simulink model "torqueBalancing"  (Simulink 8.6)
settings: Solver=FixedStepDiscrete  StartTime=0.0  StopTime=simulationTime  FixedStep=Ts  RelTol=1e-3
InitFcn:
  | initTorqueBalancing;
values from neighbouring files (symbols this model uses):
  DEMO_MOVEMENTS = false    [initTorqueBalancing.m]
  LEFT_RIGHT_FOOT_IN_CONTACT = [1 1]    [initTorqueBalancing.m]
  ON_GAZEBO = false    [initTorqueBalancing.m]
  SMOOTH_DES_COM = 1    [initTorqueBalancing.m]
  SMOOTH_DES_Q = 1    [initTorqueBalancing.m]
  Ts = 0.01    [initTorqueBalancing.m]
  USE_QP_SOLVER = 0    [initTorqueBalancing.m]
  USE_SM = true    [initTorqueBalancing.m]
  WBT_modelName = 'matlabTorqueBalancing'    [initTorqueBalancing.m]
undefined symbols (not defined in the file or in its folder): bVectorConstraints, ConstraintsMatrix, DiscIntNeverNeededParam, gain, impedencesSat, reg, ROBOT_DOF, ROBOT_DOF_FOR_SIMULINK, sat, sm
libraries: WBToolboxLibrary x55, WBCLibrary x2, simulink x2
(part 1 of 2)
settings Model: Creator=daniele  LastModifiedBy=DanielePucci
settings DataIOCC: SignalLoggingSaveFormat=Dataset
settings DebuggingCC: FcnCallInpInsideContextMsg=EnableAllAsWarning
settings SFSimCC: SimParseCustomCode=off
settings ConfigComp: CovSFcnEnable=off

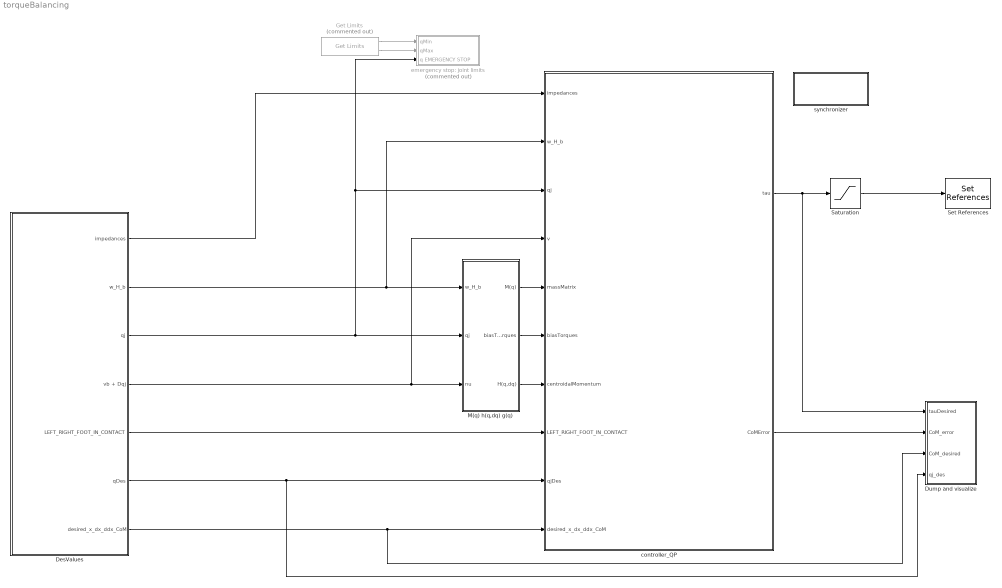
== system torqueBalancing ==
  DesValues : Subsystem  Priority=-10
  Dump and visualize : Subsystem
  Get Limits : WBToolboxLibrary/wholeBodyStates/Get Limits  Commented=on  limitsType=Position  robotName=WBT_robotName  localName=WBT_modelName  wbiFile=WBT_wbiFilename  wbiList=WBT_wbiList
  M(q) h(q,dq) g(q) : Subsystem
  Saturation : Saturate  UpperLimit=sat.torque  LowerLimit=-sat.torque
  Set References : WBToolboxLibrary/wholeBodyActuators/Set References  controlType=Torque  robotName=WBT_robotName  localName=WBT_modelName  wbiFile=WBT_wbiFilename  wbiList=WBT_wbiList
  controller_QP : Subsystem
  emergency stop: joint limits : Subsystem  Commented=on
  synchronizer : Subsystem
      mask Display: disp('SYNCHRONIZER')
  wires:
  M(q) h(q,dq) g(q)/1(M(q)) -> controller_QP/5(massMatrix)
  Get Limits/1 -> emergency stop: joint limits/1(qMin)
  Get Limits/2 -> emergency stop: joint limits/2(qMax)
  DesValues/3(qj) -> emergency stop: joint limits/3(q EMERGENCY STOP), controller_QP/3(qj), M(q) h(q,dq) g(q)/2(qj)
  M(q) h(q,dq) g(q)/2(biasTorques) -> controller_QP/6(biasTorques)
  M(q) h(q,dq) g(q)/3(H(q,dq)) -> controller_QP/7(centroidalMomentum)
  controller_QP/1("tau ") -> Saturation/1, Dump and visualize/1(tauDesired)
  controller_QP/2(CoMError) -> Dump and visualize/2(CoM_error)
  DesValues/6(qDes) -> Dump and visualize/4(qj_des), controller_QP/9(qjDes)
  DesValues/5(LEFT_RIGHT_FOOT_IN_CONTACT) -> controller_QP/8(LEFT_RIGHT_FOOT_IN_CONTACT)
  DesValues/7(desired_x_dx_ddx_CoM) -> Dump and visualize/3(CoM_desired), controller_QP/10(desired_x_dx_ddx_CoM)
  DesValues/1(impedances) -> controller_QP/1(impedances)
  Saturation/1 -> Set References/1
  DesValues/2(w_H_b) -> controller_QP/2(w_H_b), M(q) h(q,dq) g(q)/1(w_H_b)
  DesValues/4(vb + Dqj) -> controller_QP/4(v), M(q) h(q,dq) g(q)/3(nu)

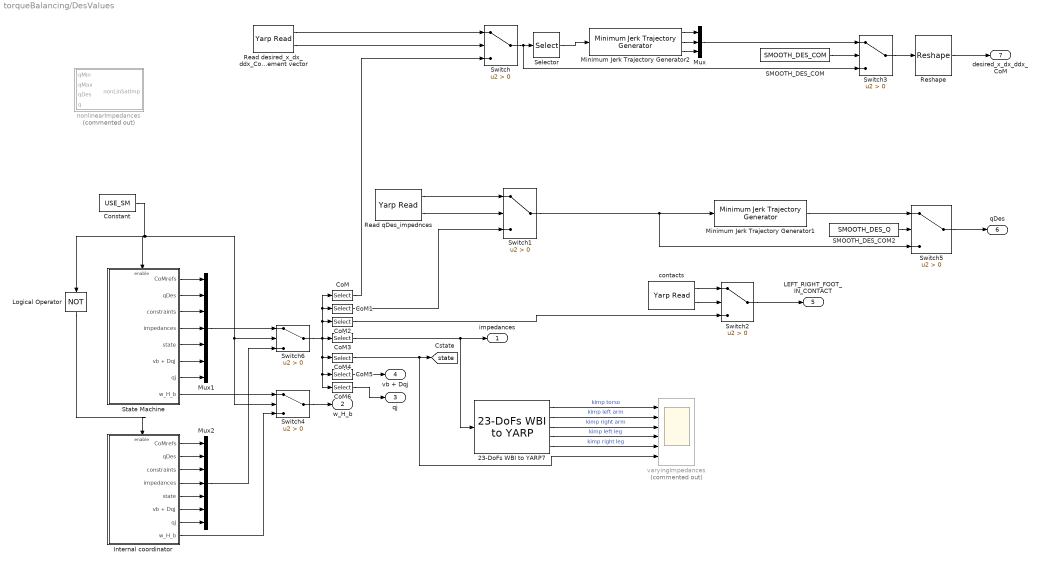
== system torqueBalancing/DesValues ==
  23-DoFs WBI to YARP7 : WBToolboxLibrary/Utilities/23-DoFs WBI to YARP
  CoM : Selector  InputPortWidth=18+4*ROBOT_DOF  IndexOptions=Index vector (dialog)  Indices=[1:9]  OutputSizes=1
  CoM1 : Selector  InputPortWidth=18+4*ROBOT_DOF  IndexOptions=Index vector (dialog)  Indices=[10:9+ROBOT_DOF]  OutputSizes=1
  CoM2 : Selector  InputPortWidth=18+4*ROBOT_DOF  IndexOptions=Index vector (dialog)  Indices=[10+ROBOT_DOF,11+ROBOT_DOF]  OutputSizes=1
  CoM3 : Selector  InputPortWidth=18+4*ROBOT_DOF  IndexOptions=Index vector (dialog)  Indices=[12+ROBOT_DOF:11+2*ROBOT_DOF]  OutputSizes=1
  CoM4 : Selector  InputPortWidth=18+4*ROBOT_DOF  IndexOptions=Index vector (dialog)  Indices=[12+2*ROBOT_DOF]  OutputSizes=1
  CoM5 : Selector  InputPortWidth=18+4*ROBOT_DOF  IndexOptions=Index vector (dialog)  Indices=[13+2*ROBOT_DOF:18+3*ROBOT_DOF]  OutputSizes=1
  CoM6 : Selector  InputPortWidth=18+4*ROBOT_DOF  IndexOptions=Index vector (dialog)  Indices=[19+3*ROBOT_DOF:18+4*ROBOT_DOF]  OutputSizes=1
  Constant : Constant  Priority=-10  Value=USE_SM
  Internal coordinator : Subsystem
  Logical Operator : Logic  Operator=NOT  AllPortsSameDT=off  OutDataTypeStr=boolean
  Minimum Jerk Trajectory Generator1 : WBToolboxLibrary/Utilities/Minimum Jerk Trajectory Generator  externalSettlingTime=off  settlingTime=references.joints.smoothingTime  sampleTime=Ts  firstDerivatives=off  secondDerivatives=off  explicitInitialValue=off
  Minimum Jerk Trajectory Generator2 : WBToolboxLibrary/Utilities/Minimum Jerk Trajectory Generator  externalSettlingTime=off  settlingTime=references.com.smoothingTime  sampleTime=Ts  firstDerivatives=on  secondDerivatives=on  explicitInitialValue=off
  Mux : Mux  Inputs=3
  Mux1 : Mux  Inputs=7
  Mux2 : Mux  Inputs=7
  Read desired_x_dx_ddx_CoM as 9 element vector : WBToolboxLibrary/Utilities/Yarp Read  portName=['/' WBT_modelName '/comDes:i']  signalSize=9  blocking=off  timestamp=off  autoconnect=off  errorOnConnection=on
  Read qDes_impednces : WBToolboxLibrary/Utilities/Yarp Read  portName=['/' WBT_modelName '/qDes:i']  signalSize=ROBOT_DOF  blocking=off  timestamp=off  autoconnect=off  errorOnConnection=on
  Reshape : Reshape  OutputDimensionality=Customize  OutputDimensions=[3,3]
  SMOOTH_DES_COM : Constant  Value=SMOOTH_DES_COM
  SMOOTH_DES_COM2 : Constant  Value=SMOOTH_DES_Q
  Selector : Selector  InputPortWidth=9  IndexOptions=Index vector (dialog)  Indices=[1 2 3]  OutputSizes=1
  State Machine : Subsystem  Priority=-100
  Switch{,1..6} (7 alike) : Switch  Criteria=u2 > Threshold
  contacts : WBToolboxLibrary/Utilities/Yarp Read  portName=['/' WBT_modelName '/constraints:i']  signalSize=2  blocking=off  timestamp=off  autoconnect=off  errorOnConnection=on
  nonlinearImpedances : Subsystem  Commented=on
  varyingImpedances : Scope  Commented=on  NumInputPorts=6
  impedances : Outport
  w_H_b : Outport  Port=2
  qj : Outport  Port=3
  vb + Dqj : Outport  Port=4
  LEFT_RIGHT_FOOT_IN_CONTACT : Outport  Port=5
  qDes : Outport  Port=6
  desired_x_dx_ddx_CoM : Outport  Port=7
  tag scope: state=global
  wires:
  Read desired_x_dx_ddx_CoM as 9 element vector/2 -> Switch/2
  Read desired_x_dx_ddx_CoM as 9 element vector/1 -> Switch/1
  Reshape/1 -> desired_x_dx_ddx_CoM/1
  Read qDes_impednces/2 -> Switch1/2
  Read qDes_impednces/1 -> Switch1/1
  contacts/2 -> Switch2/2
  contacts/1 -> Switch2/1
  CoM2/1 -> Switch2/3
  CoM/1 -> Switch/3
  CoM1/1 -> Switch1/3
  Switch/1 -> Switch3/3, Selector/1
  Selector/1 -> Minimum Jerk Trajectory Generator2/1
  Minimum Jerk Trajectory Generator2/1 -> Mux/1
  Minimum Jerk Trajectory Generator2/2 -> Mux/2
  Minimum Jerk Trajectory Generator2/3 -> Mux/3
  Mux/1 -> Switch3/1
  Switch3/1 -> Reshape/1
  SMOOTH_DES_COM/1 -> Switch3/2
  Switch2/1 -> LEFT_RIGHT_FOOT_IN_CONTACT/1
  SMOOTH_DES_COM2/1 -> Switch5/2
  Switch5/1 -> qDes/1
  Switch1/1 -> Switch5/3, Minimum Jerk Trajectory Generator1/1
  Constant/1 -> Logical Operator/1, Switch4/2, Switch6/2, State Machine/Enable
  Logical Operator/1 -> Internal coordinator/Enable
  State Machine/3(constraints) -> Mux1/3
  State Machine/2(qDes) -> Mux1/2
  State Machine/1(CoMrefs) -> Mux1/1
  Internal coordinator/1(CoMrefs) -> Mux2/1
  Internal coordinator/2(qDes) -> Mux2/2
  Internal coordinator/3(constraints) -> Mux2/3
  Mux2/1 -> Switch6/3
  Switch6/1 -> CoM6/1, CoM5/1, CoM4/1, CoM3/1, CoM/1, CoM1/1, CoM2/1
  Mux1/1 -> Switch6/1
  CoM3/1 -> 23-DoFs WBI to YARP7/1, impedances/1
  State Machine/4(impedances) -> Mux1/4
  Internal coordinator/4(impedances) -> Mux2/4
  23-DoFs WBI to YARP7/2 -> varyingImpedances/2  "kimp left arm"
  23-DoFs WBI to YARP7/4 -> varyingImpedances/4  "kimp left leg"
  23-DoFs WBI to YARP7/3 -> varyingImpedances/3  "kimp right arm"
  23-DoFs WBI to YARP7/5 -> varyingImpedances/5  "kimp right leg"
  23-DoFs WBI to YARP7/1 -> varyingImpedances/1  "kimp torso"
  State Machine/5(state) -> Mux1/5
  Internal coordinator/5(state) -> Mux2/5
  CoM4/1 -> varyingImpedances/6, [state]
  Internal coordinator/6(vb + Dqj) -> Mux2/6
  Internal coordinator/7(qj) -> Mux2/7
  State Machine/6(vb + Dqj) -> Mux1/6
  State Machine/7(qj) -> Mux1/7
  State Machine/8(w_H_b) -> Switch4/1
  Internal coordinator/8(w_H_b) -> Switch4/3
  Switch4/1 -> w_H_b/1
  CoM6/1 -> qj/1
  CoM5/1 -> vb + Dqj/1
  Minimum Jerk Trajectory Generator1/1 -> Switch5/1

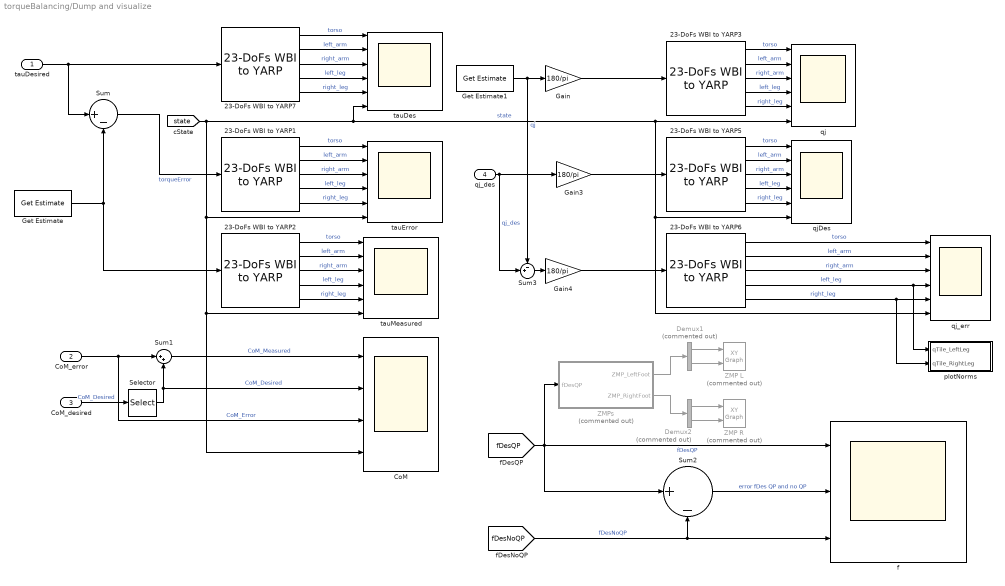
== system torqueBalancing/Dump and visualize ==
  tauDesired : Inport
  CoM_error : Inport  Port=2
  CoM_desired : Inport  Port=3
  qj_des : Inport  Port=4
  23-DoFs WBI to YARP{1..3,5..7} (6 alike) : WBToolboxLibrary/Utilities/23-DoFs WBI to YARP
  CoM : Scope  NumInputPorts=4
  Demux1 : Demux  Commented=on  Outputs=2
  Demux2 : Demux  Commented=on  Outputs=2
  Gain : Gain  Gain=180/pi
  Gain3 : Gain  Gain=180/pi
  Gain4 : Gain  Gain=180/pi
  Get Estimate : WBToolboxLibrary/wholeBodyStates/Get Estimate  estimateType=Joints Torque  robotName=WBT_robotName  localName=WBT_modelName  wbiFile=WBT_wbiFilename  wbiList=WBT_wbiList
  Get Estimate1 : WBToolboxLibrary/wholeBodyStates/Get Estimate  estimateType=Joints Position  robotName=WBT_robotName  localName=WBT_modelName  wbiFile=WBT_wbiFilename  wbiList=WBT_wbiList
  Selector : Selector  NumberOfDimensions=2  IndexOptions=Index vector (dialog),Index vector (dialog)  Indices=[1:3],1  OutputSizes=1,1
  Sum : Sum  Inputs=|+-
  Sum1 : Sum  Inputs=|++
  Sum2 : Sum  Inputs=|+-
  Sum3 : Sum  Inputs=-+|
  ZMP L : simulink/Sinks/XY Graph  Commented=on  xmin=gain.footSize(1,1)  xmax=gain.footSize(1,2)  ymin=gain.footSize(2,1)  ymax=gain.footSize(2,2)  st=-1
  ZMP R : simulink/Sinks/XY Graph  Commented=on  xmin=gain.footSize(1,1)  xmax=gain.footSize(1,2)  ymin=gain.footSize(2,1)  ymax=gain.footSize(2,2)  st=-1
  ZMPs : Subsystem  Commented=on
  f : Scope  NumInputPorts=3
  plotNorms : Subsystem
  qj : Scope  NumInputPorts=6
  qjDes : Scope  NumInputPorts=6
  qj_err : Scope  NumInputPorts=6
  tauDes : Scope  NumInputPorts=6
  tauError : Scope  NumInputPorts=6
  tauMeasured : Scope  NumInputPorts=6
  wires:
  CoM_error/1 -> Sum1/1, CoM/3  "CoM_Error"
  CoM_desired/1 -> Selector/1  "CoM_Desired"
  Sum1/1 -> CoM/1  "CoM_Measured"
  Get Estimate1/1 -> Sum3/1, Gain/1  "qj"
  Gain/1 -> 23-DoFs WBI to YARP3/1
  23-DoFs WBI to YARP3/5 -> qj/5  "right_leg"
  23-DoFs WBI to YARP3/1 -> qj/1  "torso"
  23-DoFs WBI to YARP3/2 -> qj/2  "left_arm"
  23-DoFs WBI to YARP3/4 -> qj/4  "left_leg"
  23-DoFs WBI to YARP3/3 -> qj/3  "right_arm"
  [fDesQP] -> ZMPs/1(fDesQP), Sum2/1, f/1  "fDesQP"
  ZMPs/1(ZMP_LeftFoot) -> Demux1/1
  ZMPs/2(ZMP_RightFoot) -> Demux2/1
  Demux1/1 -> ZMP L/1
  Demux1/2 -> ZMP L/2
  Demux2/1 -> ZMP R/1
  Demux2/2 -> ZMP R/2
  Sum2/1 -> f/2  "error fDes QP and no QP"
  [fDesNoQP] -> Sum2/2, f/3  "fDesNoQP"
  tauDesired/1 -> 23-DoFs WBI to YARP7/1, Sum/1
  Get Estimate/1 -> 23-DoFs WBI to YARP2/1, Sum/2
  23-DoFs WBI to YARP7/5 -> tauDes/5  "right_leg"
  23-DoFs WBI to YARP7/1 -> tauDes/1  "torso"
  23-DoFs WBI to YARP7/2 -> tauDes/2  "left_arm"
  23-DoFs WBI to YARP7/4 -> tauDes/4  "left_leg"
  23-DoFs WBI to YARP7/3 -> tauDes/3  "right_arm"
  23-DoFs WBI to YARP1/5 -> tauError/5  "right_leg"
  23-DoFs WBI to YARP1/1 -> tauError/1  "torso"
  23-DoFs WBI to YARP1/2 -> tauError/2  "left_arm"
  23-DoFs WBI to YARP1/4 -> tauError/4  "left_leg"
  23-DoFs WBI to YARP1/3 -> tauError/3  "right_arm"
  Sum/1 -> 23-DoFs WBI to YARP1/1  "torqueError"
  23-DoFs WBI to YARP2/5 -> tauMeasured/5  "right_leg"
  23-DoFs WBI to YARP2/1 -> tauMeasured/1  "torso"
  23-DoFs WBI to YARP2/2 -> tauMeasured/2  "left_arm"
  23-DoFs WBI to YARP2/4 -> tauMeasured/4  "left_leg"
  23-DoFs WBI to YARP2/3 -> tauMeasured/3  "right_arm"
  qj_des/1 -> Sum3/2, Gain3/1  "qj_des"
  Gain3/1 -> 23-DoFs WBI to YARP5/1
  23-DoFs WBI to YARP5/5 -> qjDes/5  "right_leg"
  23-DoFs WBI to YARP5/1 -> qjDes/1  "torso"
  23-DoFs WBI to YARP5/2 -> qjDes/2  "left_arm"
  23-DoFs WBI to YARP5/4 -> qjDes/4  "left_leg"
  23-DoFs WBI to YARP5/3 -> qjDes/3  "right_arm"
  Gain4/1 -> 23-DoFs WBI to YARP6/1
  23-DoFs WBI to YARP6/5 -> plotNorms/2(qTile_RightLeg), qj_err/5  "right_leg"
  23-DoFs WBI to YARP6/1 -> qj_err/1  "torso"
  23-DoFs WBI to YARP6/2 -> qj_err/2  "left_arm"
  23-DoFs WBI to YARP6/4 -> plotNorms/1(qTile_LeftLeg), qj_err/4  "left_leg"
  23-DoFs WBI to YARP6/3 -> qj_err/3  "right_arm"
  Sum3/1 -> Gain4/1
  Selector/1 -> Sum1/2, CoM/2  "CoM_Desired"
  [state] -> tauDes/6, qj_err/6, qjDes/6, qj/6, CoM/4, tauMeasured/6, tauError/6  "state"

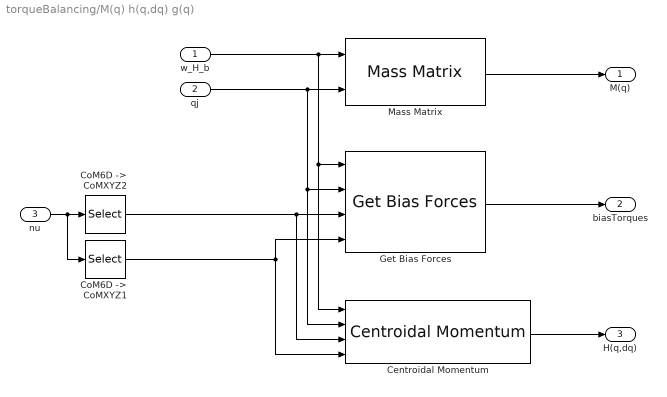
== system torqueBalancing/M(q) h(q,dq) g(q) ==
  w_H_b : Inport
  qj : Inport  Port=2
  nu : Inport  Port=3
  Centroidal Momentum : WBToolboxLibrary/wholeBodyModel/Dynamics/Centroidal Momentum  robotName=WBT_robotName  localName=WBT_modelName  wbiFile=WBT_wbiFilename  wbiList=WBT_wbiList
  "CoM6D ->  CoMXYZ1" : Selector  InputPortWidth=6+ROBOT_DOF  IndexOptions=Index vector (dialog)  Indices=[7:6+ROBOT_DOF]  OutputSizes=1
  "CoM6D ->  CoMXYZ2" : Selector  InputPortWidth=6+ROBOT_DOF  IndexOptions=Index vector (dialog)  Indices=[1 2 3 4 5 6]  OutputSizes=1
  Get Bias Forces : WBToolboxLibrary/wholeBodyModel/Dynamics/Get Bias Forces  robotName=WBT_robotName  localName=WBT_modelName  wbiFile=WBT_wbiFilename  wbiList=WBT_wbiList
  Mass Matrix : WBToolboxLibrary/wholeBodyModel/Dynamics/Mass Matrix  robotName=WBT_robotName  localName=WBT_modelName  wbiFile=WBT_wbiFilename  wbiList=WBT_wbiList
  M(q) : Outport
  biasTorques : Outport  Port=2
  H(q,dq) : Outport  Port=3
  wires:
  Mass Matrix/1 -> M(q)/1
  Centroidal Momentum/1 -> H(q,dq)/1
  Get Bias Forces/1 -> biasTorques/1
  w_H_b/1 -> Centroidal Momentum/1, Get Bias Forces/1, Mass Matrix/1
  qj/1 -> Centroidal Momentum/2, Get Bias Forces/2, Mass Matrix/2
  "CoM6D ->  CoMXYZ2"/1 -> Centroidal Momentum/3, Get Bias Forces/3
  "CoM6D ->  CoMXYZ1"/1 -> Get Bias Forces/4, Centroidal Momentum/4
  nu/1 -> "CoM6D ->  CoMXYZ1"/1, "CoM6D ->  CoMXYZ2"/1

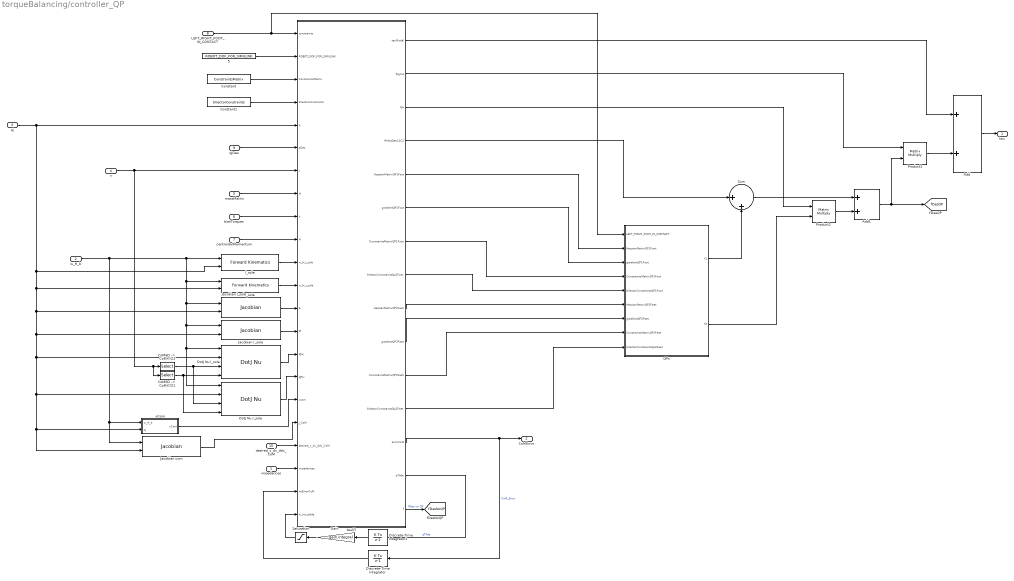
== system torqueBalancing/controller_QP ==
  impedances : Inport
  w_H_b : Inport  Port=2
  qj : Inport  Port=3
  v : Inport  Port=4
  massMatrix : Inport  Port=5
  biasTorques : Inport  Port=6
  centroidalMomentum : Inport  Port=7
  LEFT_RIGHT_FOOT_IN_CONTACT : Inport  Port=8
  qjDes : Inport  Port=9
  desired_x_dx_ddx_CoM : Inport  Port=10
  "    5" : Constant  Value=ROBOT_DOF_FOR_SIMULINK
  Add : Sum
  Add1 : Sum
  "CoM6D ->  CoMXYZ1" : Selector  InputPortWidth=6+ROBOT_DOF  IndexOptions=Index vector (dialog)  Indices=[7:6+ROBOT_DOF]  OutputSizes=1
  "CoM6D ->  CoMXYZ2" : Selector  InputPortWidth=6+ROBOT_DOF  IndexOptions=Index vector (dialog)  Indices=[1 2 3 4 5 6]  OutputSizes=1
  Constant : Constant  Value=ConstraintsMatrix
  Constant1 : Constant  Value=bVectorConstraints
  Discrete-Time Integrator : DiscreteIntegrator  InitialCondition=[0 0 0]  SampleTime=Ts  ICPrevOutput=DiscIntNeverNeededParam  ICPrevScaledInput=DiscIntNeverNeededParam
  Discrete-Time Integrator1 : DiscreteIntegrator  InitialCondition=zeros(ROBOT_DOF,1)  SampleTime=Ts  ICPrevOutput=DiscIntNeverNeededParam  ICPrevScaledInput=DiscIntNeverNeededParam
  "DotJ Nu l_sole " : WBToolboxLibrary/wholeBodyModel/Jacobians/DotJ Nu  frameName='l_sole'  robotName=WBT_robotName  localName=WBT_modelName  wbiFile=WBT_wbiFilename  wbiList=WBT_wbiList
  "DotJ Nu r_sole " : WBToolboxLibrary/wholeBodyModel/Jacobians/DotJ Nu  frameName='r_sole'  robotName=WBT_robotName  localName=WBT_modelName  wbiFile=WBT_wbiFilename  wbiList=WBT_wbiList
  Gain : Gain  Gain=gain.integral
  Jacobian com : WBToolboxLibrary/wholeBodyModel/Jacobians/Jacobian  frameName='com'  robotName=WBT_robotName  localName=WBT_modelName  wbiFile=WBT_wbiFilename  wbiList=WBT_wbiList
  Jacobian l_sole : WBToolboxLibrary/wholeBodyModel/Jacobians/Jacobian  frameName='l_sole'  robotName=WBT_robotName  localName=WBT_modelName  wbiFile=WBT_wbiFilename  wbiList=WBT_wbiList
  Jacobian r_sole : WBToolboxLibrary/wholeBodyModel/Jacobians/Jacobian  frameName='r_sole'  robotName=WBT_robotName  localName=WBT_modelName  wbiFile=WBT_wbiFilename  wbiList=WBT_wbiList
  Product1 : Product  Multiplication=Matrix(*)
  Product2 : Product  Multiplication=Matrix(*)
  QPs : Subsystem
  Saturation : Saturate  UpperLimit=sat.integral  LowerLimit=-sat.integral
  Sum : Sum  Inputs=|++
  l_sole : WBToolboxLibrary/wholeBodyModel/Kinematics/Forward Kinematics  frameName='l_sole'  robotName=WBT_robotName  localName=WBT_modelName  wbiFile=WBT_wbiFilename  wbiList=WBT_wbiList
  r_sole : WBToolboxLibrary/wholeBodyModel/Kinematics/Forward Kinematics  frameName='r_sole'  robotName=WBT_robotName  localName=WBT_modelName  wbiFile=WBT_wbiFilename  wbiList=WBT_wbiList
  "tau(f) " : MATLAB Function  TreatAsAtomicUnit=on
  xCom : Subsystem
  "tau " : Outport
  CoMError : Outport  Port=2
  tag scope: fDesNoQP=global, fDesQP=global
  wires:
  LEFT_RIGHT_FOOT_IN_CONTACT/1 -> QPs/1(LEFT_RIGHT_FOOT_IN_CONTACT), "tau(f) "/1(constraints)
  Discrete-Time Integrator/1 -> "tau(f) "/21(intErrorCoM)
  "tau(f) "/13(errorCoM) -> CoMError/1, Discrete-Time Integrator/1  "CoM_Error"
  Discrete-Time Integrator1/1 -> Gain/1
  "tau(f) "/14(qTilde) -> Discrete-Time Integrator1/1  "qTilde"
  Gain/1 -> Saturation/1
  Saturation/1 -> "tau(f) "/22(ki_int_qtilde)
  qj/1 -> l_sole/2, xCom/2(qj), Jacobian com/2, "DotJ Nu r_sole "/2, "DotJ Nu l_sole "/2, Jacobian r_sole/2, Jacobian l_sole/2, r_sole/2, "tau(f) "/5(q)
  qjDes/1 -> "tau(f) "/6(qDes)
  massMatrix/1 -> "tau(f) "/8(M)
  biasTorques/1 -> "tau(f) "/9(h)
  desired_x_dx_ddx_CoM/1 -> "tau(f) "/19(desired_x_dx_ddx_CoM)
  impedances/1 -> "tau(f) "/20(impedances)
  centroidalMomentum/1 -> "tau(f) "/10(H)
  r_sole/1 -> "tau(f) "/12(w_H_r_sole)
  l_sole/1 -> "tau(f) "/11(w_H_l_sole)
  Jacobian l_sole/1 -> "tau(f) "/13(JL)
  Jacobian r_sole/1 -> "tau(f) "/14(JR)
  Jacobian com/1 -> "tau(f) "/18(J_CoM)
  "tau(f) "/5(HessianMatrixQP1Foot) -> QPs/2(HessianMatrixQP1Foot)
  "tau(f) "/6(gradientQP1Foot) -> QPs/3(gradientQP1Foot)
  "tau(f) "/9(HessianMatrixQP2Feet) -> QPs/6(HessianMatrixQP2Feet)
  "tau(f) "/10(gradientQP2Feet) -> QPs/7(gradientQP2Feet)
  "tau(f) "/11(ConstraintsMatrixQP2Feet) -> QPs/8(ConstraintsMatrixQP2Feet)
  "tau(f) "/12(bVectorConstraintsQp2Feet) -> QPs/9(bVectorConstraintsQp2Feet)
  "tau(f) "/4(fHdotDesC1C2) -> Sum/1
  QPs/1(f1) -> Sum/2
  Product1/1 -> Add/2
  "tau(f) "/1(tauModel) -> Add/1
  Add/1 -> "tau "/1
  Add1/1 -> [fDesQP], Product1/2
  "    5"/1 -> "tau(f) "/2(ROBOT_DOF_FOR_SIMULINK)
  Constant/1 -> "tau(f) "/3(ConstraintsMatrix)
  Constant1/1 -> "tau(f) "/4(bVectorConstraints)
  "tau(f) "/7(ConstraintsMatrixQP1Foot) -> QPs/4(ConstraintsMatrixQP1Foot)
  "tau(f) "/8(bVectorConstraintsQp1Foot) -> QPs/5(bVectorConstraintsQP1Foot)
  Sum/1 -> Add1/1
  Product2/1 -> Add1/2
  "tau(f) "/3(NA) -> Product2/1
  QPs/2(f0) -> Product2/2
  "tau(f) "/2(Sigma) -> Product1/1
  "tau(f) "/15(f) -> [fDesNoQP]  "fDes no QP"
  "DotJ Nu l_sole "/1 -> "tau(f) "/15(dJLv)
  "DotJ Nu r_sole "/1 -> "tau(f) "/16(dJRv)
  xCom/1(xCom) -> "tau(f) "/17(xcom)
  v/1 -> "tau(f) "/7(v), "CoM6D ->  CoMXYZ1"/1, "CoM6D ->  CoMXYZ2"/1
  "CoM6D ->  CoMXYZ2"/1 -> "DotJ Nu r_sole "/3, "DotJ Nu l_sole "/3
  "CoM6D ->  CoMXYZ1"/1 -> "DotJ Nu r_sole "/4, "DotJ Nu l_sole "/4
  w_H_b/1 -> xCom/1(w_H_b), Jacobian com/1, r_sole/1, "DotJ Nu r_sole "/1, "DotJ Nu l_sole "/1, Jacobian r_sole/1, Jacobian l_sole/1, l_sole/1

== system torqueBalancing/emergency stop: joint limits ==
  qMin : Inport
  qMax : Inport  Port=2
  q EMERGENCY STOP : Inport  Port=3
  Assertion : Assertion
  MATLAB Function : MATLAB Function  TreatAsAtomicUnit=on
  index1 : Constant  Value=0.01  VectorParams1D=off
  wires:
  qMin/1 -> MATLAB Function/1(umin)
  qMax/1 -> MATLAB Function/2(umax)
  index1/1 -> MATLAB Function/4(tol)
  q EMERGENCY STOP/1 -> MATLAB Function/3(u)
  MATLAB Function/1(inRange) -> Assertion/1

== system torqueBalancing/synchronizer ==
  GAZEBO_SYNCHRONIZER : Subsystem  Commented=on
  Logical Operator : Logic  Operator=NOT  AllPortsSameDT=off  OutDataTypeStr=boolean
  "ON_GAZEBO " : Constant  Value=ON_GAZEBO
  REAL_TIME_SYNC : Subsystem
  wires:
  Logical Operator/1 -> REAL_TIME_SYNC/Enable
  "ON_GAZEBO "/1 -> GAZEBO_SYNCHRONIZER/Enable, Logical Operator/1

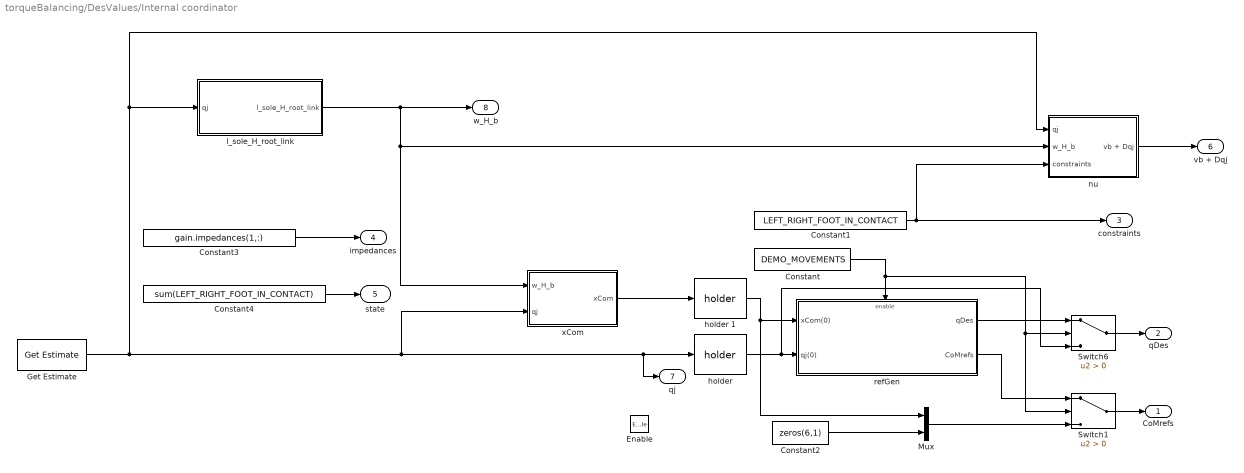
== system torqueBalancing/DesValues/Internal coordinator ==
  Enable : EnablePort
  Constant : Constant  Value=DEMO_MOVEMENTS
  Constant1 : Constant  Value=LEFT_RIGHT_FOOT_IN_CONTACT
  Constant2 : Constant  Value=zeros(6,1)
  Constant3 : Constant  Value=gain.impedances(1,:)
  Constant4 : Constant  Value=sum(LEFT_RIGHT_FOOT_IN_CONTACT)
  Get Estimate : WBToolboxLibrary/wholeBodyStates/Get Estimate  estimateType=Joints Position  robotName=WBT_robotName  localName=WBT_modelName  wbiFile=WBT_wbiFilename  wbiList=WBT_wbiList
  Mux : Mux  Inputs=2
  Switch1 : Switch  Criteria=u2 > Threshold
  Switch6 : Switch  Criteria=u2 > Threshold
  "holder " : WBToolboxLibrary/Utilities/holder 
  holder 1 : WBToolboxLibrary/Utilities/holder 
  l_sole_H_root_link : Subsystem
  nu : Subsystem
  refGen : Subsystem
  xCom : Subsystem
  CoMrefs : Outport
  qDes : Outport  Port=2
  constraints : Outport  Port=3
  impedances : Outport  Port=4
  state : Outport  Port=5
  vb + Dqj : Outport  Port=6
  qj : Outport  Port=7
  w_H_b : Outport  Port=8
  wires:
  Constant1/1 -> nu/3("constraints "), constraints/1
  Get Estimate/1 -> l_sole_H_root_link/1(qj), nu/1(qj), xCom/2(qj), "holder "/1, qj/1
  "holder "/1 -> Switch6/3, refGen/2(qj(0))
  Constant/1 -> Switch1/2, Switch6/2, refGen/Enable
  Switch6/1 -> qDes/1
  Switch1/1 -> CoMrefs/1
  refGen/1(qDes) -> Switch6/1
  refGen/2(CoMrefs) -> Switch1/1
  Mux/1 -> Switch1/3
  Constant2/1 -> Mux/2
  Constant3/1 -> impedances/1
  Constant4/1 -> state/1
  nu/1(vb + Dqj) -> vb + Dqj/1
  holder 1/1 -> Mux/1, refGen/1(xCom(0))
  l_sole_H_root_link/1(l_sole_H_root_link) -> nu/2(w_H_b), xCom/1(w_H_b), w_H_b/1
  xCom/1(xCom) -> holder 1/1

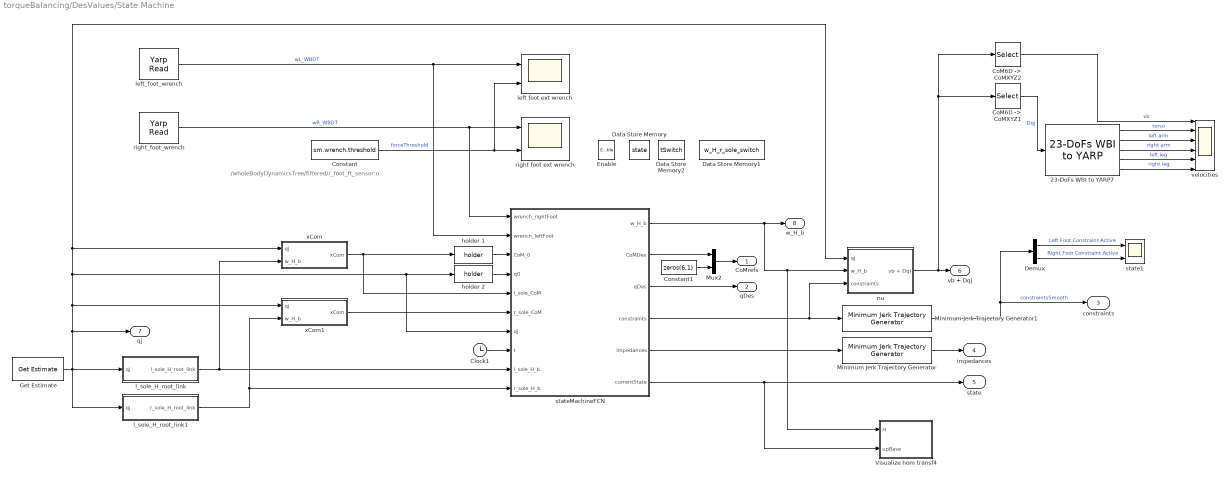
== system torqueBalancing/DesValues/State Machine ==
  note: /wholeBodyDynamicsTree/filtered/r_foot_ft_sensor:o
  Enable : EnablePort
  23-DoFs WBI to YARP7 : WBToolboxLibrary/Utilities/23-DoFs WBI to YARP
  Clock1 : Clock
  "CoM6D ->  CoMXYZ1" : Selector  InputPortWidth=ROBOT_DOF+6  IndexOptions=Index vector (dialog)  Indices=[7:ROBOT_DOF+6]  OutputSizes=1
  "CoM6D ->  CoMXYZ2" : Selector  InputPortWidth=ROBOT_DOF+6  IndexOptions=Index vector (dialog)  Indices=[1 2 3 4 5 6]  OutputSizes=1
  Constant : Constant  Value=sm.wrench.threshold
  Constant1 : Constant  Value=zeros(6,1)
  Data Store Memory : DataStoreMemory  DataStoreName=state  InitialValue=sm.stateAt0  OutDataTypeStr=double
  Data Store Memory1 : DataStoreMemory  DataStoreName=w_H_r_sole_switch  InitialValue=zeros(4)  OutDataTypeStr=double
  Data Store Memory2 : DataStoreMemory  DataStoreName=tSwitch  OutDataTypeStr=double
  Demux : Demux  Outputs=2
  Get Estimate : WBToolboxLibrary/wholeBodyStates/Get Estimate  estimateType=Joints Position  robotName=WBT_robotName  localName=WBT_modelName  wbiFile=WBT_wbiFilename  wbiList=WBT_wbiList
  Minimum Jerk Trajectory Generator : WBToolboxLibrary/Utilities/Minimum Jerk Trajectory Generator  externalSettlingTime=off  settlingTime=gain.SmoothingTimeImp  sampleTime=Ts  firstDerivatives=off  secondDerivatives=off  explicitInitialValue=off
  Minimum Jerk Trajectory Generator1 : WBToolboxLibrary/Utilities/Minimum Jerk Trajectory Generator  externalSettlingTime=off  settlingTime=smoothingTimeTransitionDynamics  sampleTime=Ts  firstDerivatives=off  secondDerivatives=off  explicitInitialValue=off
  Mux2 : Mux  Inputs=2
  Visualize hom transf4 : Subsystem
  holder 1 : WBToolboxLibrary/Utilities/holder 
  holder 2 : WBToolboxLibrary/Utilities/holder 
  l_sole_H_root_link : Subsystem
  l_sole_H_root_link1 : Subsystem
  left foot ext wrench : Scope  NumInputPorts=2
  left_foot_wrench : WBToolboxLibrary/Utilities/Yarp Read  portName='/wholeBodyDynamicsTree/left_leg/cartesianEndEffectorWrench:o'  signalSize=6  blocking=off  timestamp=off  autoconnect=on  errorOnConnection=off
  nu : Subsystem
  right foot ext wrench : Scope  NumInputPorts=2
  right_foot_wrench : WBToolboxLibrary/Utilities/Yarp Read  portName='/wholeBodyDynamicsTree/right_leg/cartesianEndEffectorWrench:o'  signalSize=6  blocking=off  timestamp=off  autoconnect=on  errorOnConnection=off
  state1 : Scope  NumInputPorts=2
  stateMachineFCN : MATLAB Function  TreatAsAtomicUnit=on
  velocities : Scope  NumInputPorts=6
  xCom : Subsystem
  xCom1 : Subsystem
  CoMrefs : Outport
  qDes : Outport  Port=2
  constraints : Outport  Port=3
  impedances : Outport  Port=4
  state : Outport  Port=5
  vb + Dqj : Outport  Port=6
  qj : Outport  Port=7
  w_H_b : Outport  Port=8
  wires:
  Constant/1 -> left foot ext wrench/2, right foot ext wrench/2  "forceThreshold"
  right_foot_wrench/1 -> right foot ext wrench/1, stateMachineFCN/1(wrench_rightFoot)  "wR_WBDT"
  Get Estimate/1 -> l_sole_H_root_link1/1(qj), l_sole_H_root_link/1(qj), nu/1(qj), xCom/1(qj), stateMachineFCN/7(qj), holder 2/1, xCom1/1(qj), qj/1
  xCom/1(xCom) -> stateMachineFCN/5(l_sole_CoM), holder 1/1
  holder 1/1 -> stateMachineFCN/3(CoM_0)
  holder 2/1 -> stateMachineFCN/4(q0)
  Clock1/1 -> stateMachineFCN/8(t)
  stateMachineFCN/3(qDes) -> qDes/1
  stateMachineFCN/2(CoMDes) -> Mux2/1
  Mux2/1 -> CoMrefs/1
  Constant1/1 -> Mux2/2
  stateMachineFCN/5(impedances) -> Minimum Jerk Trajectory Generator/1
  stateMachineFCN/6(currentState) -> state/1, Visualize hom transf4/2(upBase)
  Minimum Jerk Trajectory Generator1/1 -> Demux/1, constraints/1  "constraintsSmooth"
  stateMachineFCN/4(constraints) -> Minimum Jerk Trajectory Generator1/1, nu/3("constraints ")
  Demux/1 -> state1/1  "Left Foot Constraint Active"
  Demux/2 -> state1/2  "Right Foot Constraint Active"
  left_foot_wrench/1 -> stateMachineFCN/2(wrench_leftFoot), left foot ext wrench/1  "wL_WBDT"
  stateMachineFCN/1(w_H_b) -> nu/2(w_H_b), Visualize hom transf4/1(H), w_H_b/1
  l_sole_H_root_link/1(l_sole_H_root_link) -> stateMachineFCN/9(l_sole_H_b), xCom/2(w_H_b)
  l_sole_H_root_link1/1(r_sole_H_root_link) -> stateMachineFCN/10(r_sole_H_b), xCom1/2(w_H_b)
  xCom1/1(xCom) -> stateMachineFCN/6(r_sole_CoM)
  nu/1(vb + Dqj) -> "CoM6D ->  CoMXYZ1"/1, "CoM6D ->  CoMXYZ2"/1, vb + Dqj/1
  Minimum Jerk Trajectory Generator/1 -> impedances/1
  "CoM6D ->  CoMXYZ2"/1 -> velocities/1  "vb"
  "CoM6D ->  CoMXYZ1"/1 -> 23-DoFs WBI to YARP7/1  "Dqj"
  23-DoFs WBI to YARP7/1 -> velocities/2  "torso"
  23-DoFs WBI to YARP7/2 -> velocities/3  "left arm"
  23-DoFs WBI to YARP7/3 -> velocities/4  "right arm"
  23-DoFs WBI to YARP7/4 -> velocities/5  "left leg"
  23-DoFs WBI to YARP7/5 -> velocities/6  "right leg"

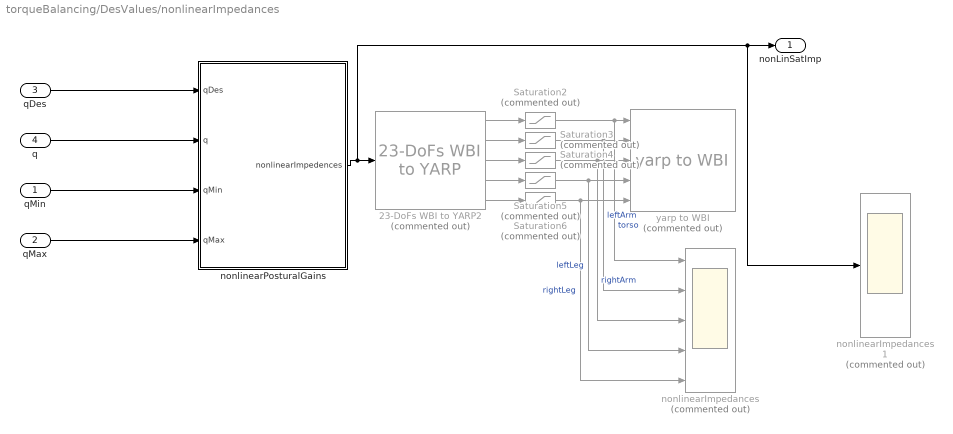
== system torqueBalancing/DesValues/nonlinearImpedances ==
  qMin : Inport
  qMax : Inport  Port=2
  qDes : Inport  Port=3
  q : Inport  Port=4
  23-DoFs WBI to YARP2 : WBCLibrary/Utilities/23-DoFs WBI to YARP  Commented=on
  Saturation2 : Saturate  Commented=on  UpperLimit=impedencesSat(1)  LowerLimit=0  SampleTime=Ts
  Saturation3 : Saturate  Commented=on  UpperLimit=impedencesSat(2)  LowerLimit=0  SampleTime=Ts
  Saturation4 : Saturate  Commented=on  UpperLimit=impedencesSat(2)  LowerLimit=0  SampleTime=Ts
  Saturation5 : Saturate  Commented=on  UpperLimit=impedencesSat(3)  LowerLimit=0  SampleTime=Ts
  Saturation6 : Saturate  Commented=on  UpperLimit=impedencesSat(3)  LowerLimit=0  SampleTime=Ts
  nonlinearImpedances : Scope  Commented=on  NumInputPorts=5
  nonlinearImpedances1 : Scope  Commented=on
  "nonlinearPosturalGains " : MATLAB Function  TreatAsAtomicUnit=on
  yarp to WBI : WBCLibrary/Utilities/yarp to WBI  Commented=on
  nonLinSatImp : Outport
  wires:
  23-DoFs WBI to YARP2/1 -> Saturation2/1
  23-DoFs WBI to YARP2/2 -> Saturation3/1
  23-DoFs WBI to YARP2/3 -> Saturation4/1
  23-DoFs WBI to YARP2/5 -> Saturation6/1
  "nonlinearPosturalGains "/1(nonlinearImpedences) -> nonlinearImpedances1/1, nonLinSatImp/1, 23-DoFs WBI to YARP2/1
  qMin/1 -> "nonlinearPosturalGains "/3(qMin)
  qMax/1 -> "nonlinearPosturalGains "/4(qMax)
  q/1 -> "nonlinearPosturalGains "/2(q)
  Saturation6/1 -> nonlinearImpedances/5, yarp to WBI/5  "rightLeg"
  Saturation4/1 -> nonlinearImpedances/3, yarp to WBI/3  "rightArm"
  Saturation5/1 -> nonlinearImpedances/4, yarp to WBI/4  "leftLeg"
  Saturation3/1 -> nonlinearImpedances/2, yarp to WBI/2  "leftArm"
  Saturation2/1 -> nonlinearImpedances/1, yarp to WBI/1  "torso"
  23-DoFs WBI to YARP2/4 -> Saturation5/1
  qDes/1 -> "nonlinearPosturalGains "/1(qDes)

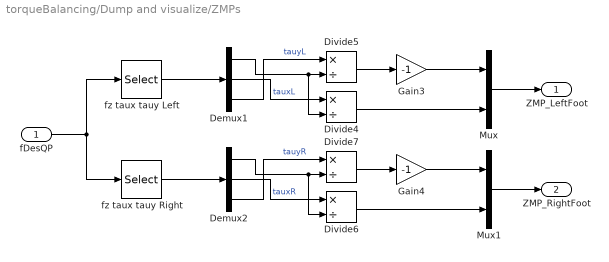
== system torqueBalancing/Dump and visualize/ZMPs ==
  fDesQP : Inport
  Demux1 : Demux  Outputs=3
  Demux2 : Demux  Outputs=3
  Divide{4..7} (4 alike) : Product  Inputs=*/
  Gain3 : Gain  Gain=-1
  Gain4 : Gain  Gain=-1
  Mux : Mux  Inputs=2
  Mux1 : Mux  Inputs=2
  fz taux tauy Left : Selector  InputPortWidth=12  IndexOptions=Index vector (dialog)  Indices=[3 4 5]  OutputSizes=1
  fz taux tauy Right : Selector  InputPortWidth=12  IndexOptions=Index vector (dialog)  Indices=[9 10 11]  OutputSizes=1
  ZMP_LeftFoot : Outport
  ZMP_RightFoot : Outport  Port=2
  wires:
  fz taux tauy Left/1 -> Demux1/1
  Demux1/1 -> Divide4/2, Divide5/2
  Divide7/1 -> Gain4/1
  Divide4/1 -> Mux/2
  Divide5/1 -> Gain3/1
  fz taux tauy Right/1 -> Demux2/1
  Demux2/1 -> Divide6/2, Divide7/2
  fDesQP/1 -> fz taux tauy Left/1, fz taux tauy Right/1
  Gain3/1 -> Mux/1
  Mux/1 -> ZMP_LeftFoot/1
  Divide6/1 -> Mux1/2
  Gain4/1 -> Mux1/1
  Mux1/1 -> ZMP_RightFoot/1
  Demux1/2 -> Divide4/1  "tauxL"
  Demux1/3 -> Divide5/1  "tauyL"
  Demux2/2 -> Divide6/1  "tauxR"
  Demux2/3 -> Divide7/1  "tauyR"

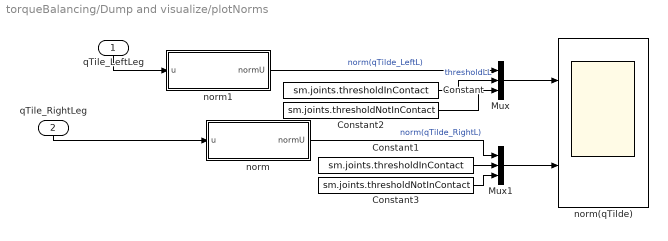
== system torqueBalancing/Dump and visualize/plotNorms ==
  qTile_LeftLeg : Inport
  qTile_RightLeg : Inport  Port=2
  Constant : Constant  Value=sm.joints.thresholdInContact
  Constant1 : Constant  Value=sm.joints.thresholdInContact
  Constant2 : Constant  Value=sm.joints.thresholdNotInContact
  Constant3 : Constant  Value=sm.joints.thresholdNotInContact
  Mux : Mux  Inputs=3
  Mux1 : Mux  Inputs=3
  norm : MATLAB Function  TreatAsAtomicUnit=on
  norm(qTilde) : Scope  NumInputPorts=2
  norm1 : MATLAB Function  TreatAsAtomicUnit=on
  wires:
  Constant/1 -> Mux/2  "thresholdLL"
  qTile_LeftLeg/1 -> norm1/1(u)
  qTile_RightLeg/1 -> norm/1(u)
  norm/1(normU) -> Mux1/1  "norm(qTilde_RightL)"
  norm1/1(normU) -> Mux/1  "norm(qTilde_LeftL)"
  Mux/1 -> norm(qTilde)/1
  Mux1/1 -> norm(qTilde)/2
  Constant2/1 -> Mux/3
  Constant1/1 -> Mux1/2
  Constant3/1 -> Mux1/3

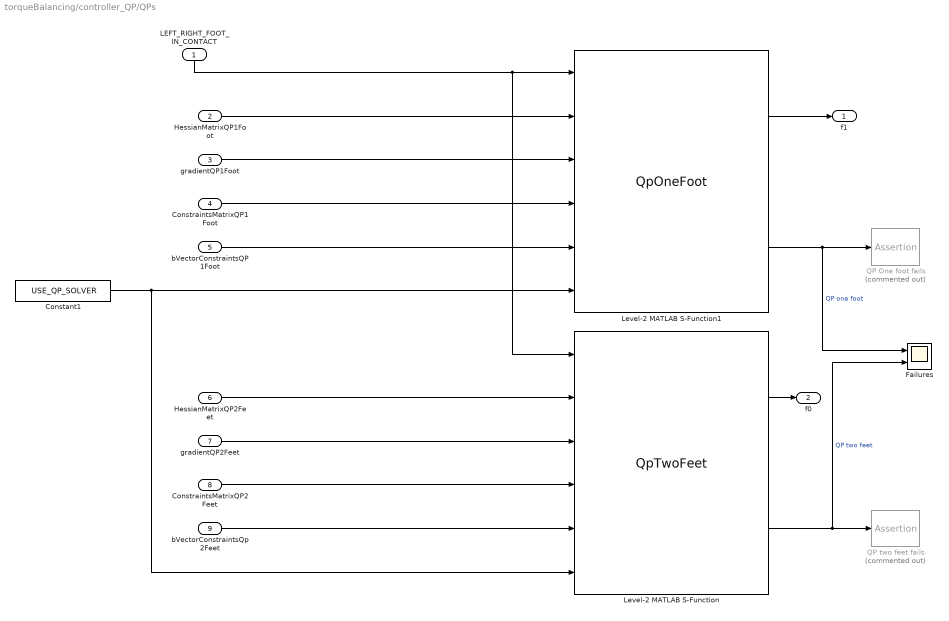
== system torqueBalancing/controller_QP/QPs ==
  LEFT_RIGHT_FOOT_IN_CONTACT : Inport
  HessianMatrixQP1Foot : Inport  Port=2
  gradientQP1Foot : Inport  Port=3
  ConstraintsMatrixQP1Foot : Inport  Port=4
  bVectorConstraintsQP1Foot : Inport  Port=5
  HessianMatrixQP2Feet : Inport  Port=6
  gradientQP2Feet : Inport  Port=7
  ConstraintsMatrixQP2Feet : Inport  Port=8
  bVectorConstraintsQp2Feet : Inport  Port=9
  Constant1 : Constant  Value=USE_QP_SOLVER
  Failures : Scope  NumInputPorts=2
  Level-2 MATLAB S-Function : M-S-Function  FunctionName=QpTwoFeet
  Level-2 MATLAB S-Function1 : M-S-Function  FunctionName=QpOneFoot
  QP One foot fails : Assertion  Commented=on
  QP two feet fails : Assertion  Commented=on
  f1 : Outport
  f0 : Outport  Port=2
  wires:
  LEFT_RIGHT_FOOT_IN_CONTACT/1 -> Level-2 MATLAB S-Function/1, Level-2 MATLAB S-Function1/1
  gradientQP2Feet/1 -> Level-2 MATLAB S-Function/3
  HessianMatrixQP1Foot/1 -> Level-2 MATLAB S-Function1/2
  ConstraintsMatrixQP2Feet/1 -> Level-2 MATLAB S-Function/4
  gradientQP1Foot/1 -> Level-2 MATLAB S-Function1/3
  HessianMatrixQP2Feet/1 -> Level-2 MATLAB S-Function/2
  Level-2 MATLAB S-Function/1 -> f0/1
  bVectorConstraintsQp2Feet/1 -> Level-2 MATLAB S-Function/5
  Level-2 MATLAB S-Function1/1 -> f1/1
  ConstraintsMatrixQP1Foot/1 -> Level-2 MATLAB S-Function1/4
  bVectorConstraintsQP1Foot/1 -> Level-2 MATLAB S-Function1/5
  Level-2 MATLAB S-Function/2 -> Failures/2, QP two feet fails/1  "QP two feet"
  Constant1/1 -> Level-2 MATLAB S-Function/6, Level-2 MATLAB S-Function1/6
  Level-2 MATLAB S-Function1/2 -> Failures/1, QP One foot fails/1  "QP one foot"

== system torqueBalancing/controller_QP/xCom ==
  w_H_b : Inport
  qj : Inport  Port=2
  "CoM6D ->  CoMXYZ2" : Selector  NumberOfDimensions=2  InputPortWidth=7  IndexOptions=Index vector (dialog),Index vector (dialog)  Indices=[1 2 3],[4]  OutputSizes=1,1
  com : WBToolboxLibrary/wholeBodyModel/Kinematics/Forward Kinematics  frameName='com'  robotName=WBT_robotName  localName=WBT_modelName  wbiFile=WBT_wbiFilename  wbiList=WBT_wbiList
  xCom : Outport
  wires:
  qj/1 -> com/2
  "CoM6D ->  CoMXYZ2"/1 -> xCom/1
  com/1 -> "CoM6D ->  CoMXYZ2"/1
  w_H_b/1 -> com/1

== system torqueBalancing/synchronizer/GAZEBO_SYNCHRONIZER ==
  Enable : EnablePort
  Simulator Synchronizer : WBToolboxLibrary/Utilities/Simulator Synchronizer  period=Ts  serverPortName='/clock/rpc'  clientPortName='/WBT_synchronizer/rpc:o'

== system torqueBalancing/synchronizer/REAL_TIME_SYNC ==
  Enable : EnablePort
  Real Time Synchronizer : WBToolboxLibrary/Utilities/Real Time Synchronizer  period=Ts

== system torqueBalancing/DesValues/Internal coordinator/l_sole_H_root_link ==
  qj : Inport
  Constant5 : Constant  Value=eye(4)
  Constant6 : Constant  Value=eye(4)
  Inv\* : Product  Inputs=/*  Multiplication=Matrix(*)
  l_sole : WBToolboxLibrary/wholeBodyModel/Kinematics/Forward Kinematics  frameName='l_sole'  robotName=WBT_robotName  localName=WBT_modelName  wbiFile=WBT_wbiFilename  wbiList=WBT_wbiList
  root_link : WBToolboxLibrary/wholeBodyModel/Kinematics/Forward Kinematics  frameName='root_link'  robotName=WBT_robotName  localName=WBT_modelName  wbiFile=WBT_wbiFilename  wbiList=WBT_wbiList
  l_sole_H_root_link : Outport
  wires:
  Constant5/1 -> l_sole/1
  Inv\*/1 -> l_sole_H_root_link/1  "l_sole_H_root_link"
  l_sole/1 -> Inv\*/1
  Constant6/1 -> root_link/1
  qj/1 -> l_sole/2, root_link/2
  root_link/1 -> Inv\*/2

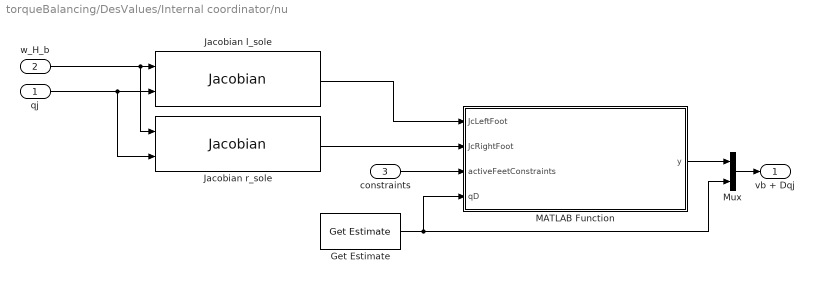
== system torqueBalancing/DesValues/Internal coordinator/nu ==
  qj : Inport
  w_H_b : Inport  Port=2
  "constraints " : Inport  Port=3
  Get Estimate : WBToolboxLibrary/wholeBodyStates/Get Estimate  estimateType=Joints Velocity  robotName=WBT_robotName  localName=WBT_modelName  wbiFile=WBT_wbiFilename  wbiList=WBT_wbiList
  Jacobian l_sole : WBToolboxLibrary/wholeBodyModel/Jacobians/Jacobian  frameName='l_sole'  robotName=WBT_robotName  localName=WBT_modelName  wbiFile=WBT_wbiFilename  wbiList=WBT_wbiList
  Jacobian r_sole : WBToolboxLibrary/wholeBodyModel/Jacobians/Jacobian  frameName='r_sole'  robotName=WBT_robotName  localName=WBT_modelName  wbiFile=WBT_wbiFilename  wbiList=WBT_wbiList
  MATLAB Function : MATLAB Function  TreatAsAtomicUnit=on
  Mux : Mux  Inputs=2
  vb + Dqj : Outport
  wires:
  Get Estimate/1 -> MATLAB Function/4(qD), Mux/2
  Mux/1 -> vb + Dqj/1
  Jacobian r_sole/1 -> MATLAB Function/2(JcRightFoot)
  "constraints "/1 -> MATLAB Function/3(activeFeetConstraints)
  MATLAB Function/1(y) -> Mux/1
  Jacobian l_sole/1 -> MATLAB Function/1(JcLeftFoot)
  qj/1 -> Jacobian r_sole/2, Jacobian l_sole/2
  w_H_b/1 -> Jacobian r_sole/1, Jacobian l_sole/1

== system torqueBalancing/DesValues/Internal coordinator/refGen ==
  xCom(0) : Inport
  qj(0) : Inport  Port=2
  Enable : EnablePort
  Clock1 : Clock
  refGenFCN : MATLAB Function  TreatAsAtomicUnit=on
  qDes : Outport
  CoMrefs : Outport  Port=2
  wires:
  refGenFCN/2(desired_x_dx_ddx_CoM) -> CoMrefs/1
  xCom(0)/1 -> refGenFCN/1(xCom0)
  Clock1/1 -> refGenFCN/3(t)
  qj(0)/1 -> refGenFCN/2(q0)
  refGenFCN/1(qDes) -> qDes/1

== system torqueBalancing/DesValues/Internal coordinator/xCom ==
  w_H_b : Inport
  qj : Inport  Port=2
  "CoM6D ->  CoMXYZ2" : Selector  NumberOfDimensions=2  InputPortWidth=7  IndexOptions=Index vector (dialog),Index vector (dialog)  Indices=[1 2 3],[4]  OutputSizes=1,1
  com : WBToolboxLibrary/wholeBodyModel/Kinematics/Forward Kinematics  frameName='com'  robotName=WBT_robotName  localName=WBT_modelName  wbiFile=WBT_wbiFilename  wbiList=WBT_wbiList
  xCom : Outport
  wires:
  qj/1 -> com/2
  "CoM6D ->  CoMXYZ2"/1 -> xCom/1
  com/1 -> "CoM6D ->  CoMXYZ2"/1
  w_H_b/1 -> com/1

== system torqueBalancing/DesValues/State Machine/Visualize hom transf4 ==
  H : Inport
  upBase : Inport  Port=2
  "CoM6D ->  CoMXYZ1" : Selector  NumberOfDimensions=2  InputPortWidth=7  IndexOptions=Index vector (dialog),Index vector (dialog)  Indices=[1 2 3],[1 2 3]  OutputSizes=1,1
  "CoM6D ->  CoMXYZ2" : Selector  NumberOfDimensions=2  InputPortWidth=7  IndexOptions=Index vector (dialog),Index vector (dialog)  Indices=[1 2 3],[4]  OutputSizes=1,1
  Hom : Scope  NumInputPorts=2
  R : Scope  NumInputPorts=2
  p : Scope  NumInputPorts=2
  wires:
  "CoM6D ->  CoMXYZ1"/1 -> R/1
  "CoM6D ->  CoMXYZ2"/1 -> p/1
  H/1 -> "CoM6D ->  CoMXYZ2"/1, Hom/1, "CoM6D ->  CoMXYZ1"/1
  upBase/1 -> p/2, R/2, Hom/2

== system torqueBalancing/DesValues/State Machine/l_sole_H_root_link ==
  qj : Inport
  Constant5 : Constant  Value=eye(4)
  Constant6 : Constant  Value=eye(4)
  Inv\* : Product  Inputs=/*  Multiplication=Matrix(*)
  l_sole : WBToolboxLibrary/wholeBodyModel/Kinematics/Forward Kinematics  frameName='l_sole'  robotName=WBT_robotName  localName=WBT_modelName  wbiFile=WBT_wbiFilename  wbiList=WBT_wbiList
  root_link : WBToolboxLibrary/wholeBodyModel/Kinematics/Forward Kinematics  frameName='root_link'  robotName=WBT_robotName  localName=WBT_modelName  wbiFile=WBT_wbiFilename  wbiList=WBT_wbiList
  l_sole_H_root_link : Outport
  wires:
  Constant5/1 -> l_sole/1
  Inv\*/1 -> l_sole_H_root_link/1  "l_sole_H_root_link"
  l_sole/1 -> Inv\*/1
  Constant6/1 -> root_link/1
  qj/1 -> l_sole/2, root_link/2
  root_link/1 -> Inv\*/2

== system torqueBalancing/DesValues/State Machine/l_sole_H_root_link1 ==
  qj : Inport
  Constant5 : Constant  Value=eye(4)
  Constant6 : Constant  Value=eye(4)
  Inv\* : Product  Inputs=/*  Multiplication=Matrix(*)
  r_sole : WBToolboxLibrary/wholeBodyModel/Kinematics/Forward Kinematics  frameName='r_sole'  robotName=WBT_robotName  localName=WBT_modelName  wbiFile=WBT_wbiFilename  wbiList=WBT_wbiList
  root_link : WBToolboxLibrary/wholeBodyModel/Kinematics/Forward Kinematics  frameName='root_link'  robotName=WBT_robotName  localName=WBT_modelName  wbiFile=WBT_wbiFilename  wbiList=WBT_wbiList
  r_sole_H_root_link : Outport
  wires:
  Constant5/1 -> r_sole/1
  Inv\*/1 -> r_sole_H_root_link/1
  r_sole/1 -> Inv\*/1
  Constant6/1 -> root_link/1
  qj/1 -> r_sole/2, root_link/2
  root_link/1 -> Inv\*/2

== system torqueBalancing/DesValues/State Machine/nu ==
  qj : Inport
  w_H_b : Inport  Port=2
  "constraints " : Inport  Port=3
  Get Estimate : WBToolboxLibrary/wholeBodyStates/Get Estimate  estimateType=Joints Velocity  robotName=WBT_robotName  localName=WBT_modelName  wbiFile=WBT_wbiFilename  wbiList=WBT_wbiList
  Jacobian l_sole : WBToolboxLibrary/wholeBodyModel/Jacobians/Jacobian  frameName='l_sole'  robotName=WBT_robotName  localName=WBT_modelName  wbiFile=WBT_wbiFilename  wbiList=WBT_wbiList
  Jacobian r_sole : WBToolboxLibrary/wholeBodyModel/Jacobians/Jacobian  frameName='r_sole'  robotName=WBT_robotName  localName=WBT_modelName  wbiFile=WBT_wbiFilename  wbiList=WBT_wbiList
  MATLAB Function : MATLAB Function  TreatAsAtomicUnit=on
  Mux : Mux  Inputs=2
  vb + Dqj : Outport
  wires:
  Get Estimate/1 -> MATLAB Function/4(qD), Mux/2
  Mux/1 -> vb + Dqj/1
  Jacobian r_sole/1 -> MATLAB Function/2(JcRightFoot)
  "constraints "/1 -> MATLAB Function/3(activeFeetConstraints)
  MATLAB Function/1(y) -> Mux/1
  Jacobian l_sole/1 -> MATLAB Function/1(JcLeftFoot)
  qj/1 -> Jacobian r_sole/2, Jacobian l_sole/2
  w_H_b/1 -> Jacobian r_sole/1, Jacobian l_sole/1

== system torqueBalancing/DesValues/State Machine/xCom ==
  qj : Inport
  w_H_b : Inport  Port=2
  "CoM6D ->  CoMXYZ2" : Selector  NumberOfDimensions=2  InputPortWidth=7  IndexOptions=Index vector (dialog),Index vector (dialog)  Indices=[1 2 3],[4]  OutputSizes=1,1
  com : WBToolboxLibrary/wholeBodyModel/Kinematics/Forward Kinematics  frameName='com'  robotName=WBT_robotName  localName=WBT_modelName  wbiFile=WBT_wbiFilename  wbiList=WBT_wbiList
  xCom : Outport
  wires:
  qj/1 -> com/2
  "CoM6D ->  CoMXYZ2"/1 -> xCom/1
  com/1 -> "CoM6D ->  CoMXYZ2"/1
  w_H_b/1 -> com/1

== system torqueBalancing/DesValues/State Machine/xCom1 ==
  qj : Inport
  w_H_b : Inport  Port=2
  "CoM6D ->  CoMXYZ2" : Selector  NumberOfDimensions=2  InputPortWidth=7  IndexOptions=Index vector (dialog),Index vector (dialog)  Indices=[1 2 3],[4]  OutputSizes=1,1
  com : WBToolboxLibrary/wholeBodyModel/Kinematics/Forward Kinematics  frameName='com'  robotName=WBT_robotName  localName=WBT_modelName  wbiFile=WBT_wbiFilename  wbiList=WBT_wbiList
  xCom : Outport
  wires:
  qj/1 -> com/2
  "CoM6D ->  CoMXYZ2"/1 -> xCom/1
  com/1 -> "CoM6D ->  CoMXYZ2"/1
  w_H_b/1 -> com/1

== matlab function DesValues/Internal coordinator/nu/MATLAB Function ==
  data: JcLeftFoot input double; JcRightFoot input double; activeFeetConstraints input double; y output double; qD input double; reg parameter double
function y = fcn(JcLeftFoot,JcRightFoot,activeFeetConstraints,qD,reg)
%#codegen

Jc = [activeFeetConstraints(1)*JcLeftFoot;
      activeFeetConstraints(2)*JcRightFoot];

pinvJb = (Jc(:,1:6)'*Jc(:,1:6) + reg.pinvDampVb*eye(6))\Jc(:,1:6)';  
  
% pinvJb = pinv(Jc(:,1:6));

y = -pinvJb*Jc(:,7:end)*qD;

== matlab function DesValues/Internal coordinator/refGen/refGenFCN ==
  data: xCom0 input double; qDes output double; q0 input double; t input double; references parameter double; desired_x_dx_ddx_CoM output double
function [qDes,desired_x_dx_ddx_CoM] = refGenFCN(xCom0,q0,t,references)
%#codegen

[qDes,desired_x_dx_ddx_CoM] = refGen(xCom0,q0,t,references);

== matlab function DesValues/State Machine/nu/MATLAB Function ==
  data: JcLeftFoot input double; JcRightFoot input double; activeFeetConstraints input double; y output double; qD input double; reg parameter double
function y = fcn(JcLeftFoot,JcRightFoot,activeFeetConstraints,qD,reg)
%#codegen

Jc = [activeFeetConstraints(1)*JcLeftFoot;
      activeFeetConstraints(2)*JcRightFoot];

pinvJb = (Jc(:,1:6)'*Jc(:,1:6) + reg.pinvDampVb*eye(6))\Jc(:,1:6)';  
  
% pinvJb = pinv(Jc(:,1:6));

y = -pinvJb*Jc(:,7:end)*qD;

== matlab function DesValues/State Machine/stateMachineFCN ==
  data: wrench_rightFoot input double; wrench_leftFoot input double; w_H_b output double; CoMDes output double; qDes output double; constraints output double; state data_store_memory double; CoM_0 input double; q0 input double; l_sole_CoM input double; r_sole_CoM input double; qj input double; t input double; l_sole_H_b input double; r_sole_H_b input double; tSwitch data_store_memory double; sm parameter double; impedances output double; gain parameter double; currentState output double; w_H_r_sole_switch data_store_memory double
function [w_H_b, CoMDes,qDes,constraints,impedances,currentState] = ...
    stateMachineFCN(wrench_rightFoot,wrench_leftFoot,CoM_0, q0, l_sole_CoM,r_sole_CoM,qj, t, l_sole_H_b, r_sole_H_b, sm,gain)
%#codegen
 
[CoMDes,qDes,constraints, currentState,impedances,w_H_b] = ...
    stateMachine(CoM_0, q0, l_sole_CoM,r_sole_CoM,qj, t, wrench_rightFoot,wrench_leftFoot,l_sole_H_b, r_sole_H_b, sm,gain);

== matlab function DesValues/nonlinearImpedances/nonlinearPosturalGains  ==
  data: qDes input double; nonlinearImpedences output double; q input double; qMin input double; qMax input double; gain parameter double
function nonlinearImpedences = fcn(qDes,q,qMin,qMax,gain)
    %#codegen
    impedences_at_0     = gain.impedances;
    increasingRatesImp  = (gain.increasingRatesImp)';
    qTildeMax           = gain.qTildeMax;

    tp =  pi./(2*(qMax-qDes));
    tn = -pi./(2*(qMin-qDes));

    
    qTilde = q - qDes;
            
    nonlinearImpedences = (impedences_at_0'   + increasingRatesImp.*tan(pi.*qTilde./(2*qTildeMax)).^2)';
%                                                increasingRatesImp.*tan((tp.*stepFcn(qTilde) + tn.*stepFcn(-qTilde)).*qTilde).^2)';
                                           
end

function y = stepFcn(x) 
   %#codegen
   y = x > 0; 
end

== matlab function Dump and visualize/plotNorms/norm ==
  data: u input double; normU output double
function normU = fcn(u)
%#codegen

normU = norm(u);

== matlab function Dump and visualize/plotNorms/norm1 ==
  data: u input double; normU output double
function normU = fcn(u)
%#codegen

normU = norm(u);
